simulink library "transformer_lib"  (Simulink 8.1)
settings: Solver=ode45  StartTime=0.0  StopTime=10.0  RelTol=1e-3
undefined symbols (not defined in the file): D1, Delta, Rating, Ts
libraries: powerlib x4, powerlib_extras x2, transformer_lib x1
settings Model: Creator=mi24996  LastModifiedBy=ed12083

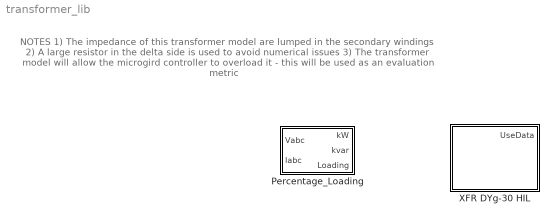
== system transformer_lib ==
  note: NOTES
      | 1) The impedance of this transformer model are lumped in the secondary windings
      | 2) A large resistor in the delta side is used to avoid numerical issues
      | 3) The transformer model will allow the microgird controller to overload it - this will be used as an evaluation metric
  Percentage_Loading : Subsystem  mask(Percentage Loading Block){kVA=Rating}
      mask help:
      | This block calculates the percentage loading of the
      | tranformer in reference to its nameplate data.
  XFR DYg-30 HIL : Subsystem  mask(Transformers){Rating=225, Vp=4160, Vs=208, Z=5.18, XR=2.5}
      mask prompts: Rating "Rating [kVA]"; Vp "Primary Voltage [VRMSLL]"; Vs "Secondary Voltage [VRMSLL]"; Z "Impedance, Z [%]"; XR "X/R Ratio"
      mask help:
      | The distribution transformer is implemented using three single-phase transformers connected D/Ygrounded with a negative 30 degrees angular displacement, and operated with fixed turn ratios.
      | The connectivity convention of this block is as follows: ABC indicates the “primary” or high voltage side, and the abc indicates the “secondary” or low voltage side.

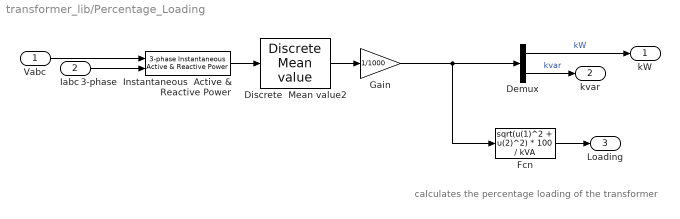
== system transformer_lib/Percentage_Loading ==
  note: calculates the percentage loading of the transformer
  Vabc : Inport
  Iabc : Inport  Port=2
  3-phase  Instantaneous  Active & Reactive Power : powerlib_extras/Measurements/3-phase  Instantaneous  Active & Reactive Power
  Demux : Demux  Outputs=2
  Discrete  Mean value2 : powerlib_extras/Discrete Measurements/Discrete  Mean value  Freq=60  Vinit=0  Ts=Ts
  Fcn : Fcn  Expr=sqrt(u(1)^2 + u(2)^2) * 100 / kVA
  Gain : Gain  Gain=1/1000
  kW : Outport
  kvar : Outport  Port=2
  Loading : Outport  Port=3
  wires:
  Fcn/1 -> Loading/1
  Demux/2 -> kvar/1  "kvar"
  Demux/1 -> kW/1  "kW"
  Iabc/1 -> 3-phase  Instantaneous  Active & Reactive Power/2
  Vabc/1 -> 3-phase  Instantaneous  Active & Reactive Power/1
  Discrete  Mean value2/1 -> Gain/1
  3-phase  Instantaneous  Active & Reactive Power/1 -> Discrete  Mean value2/1
  Gain/1 -> Demux/1, Fcn/1

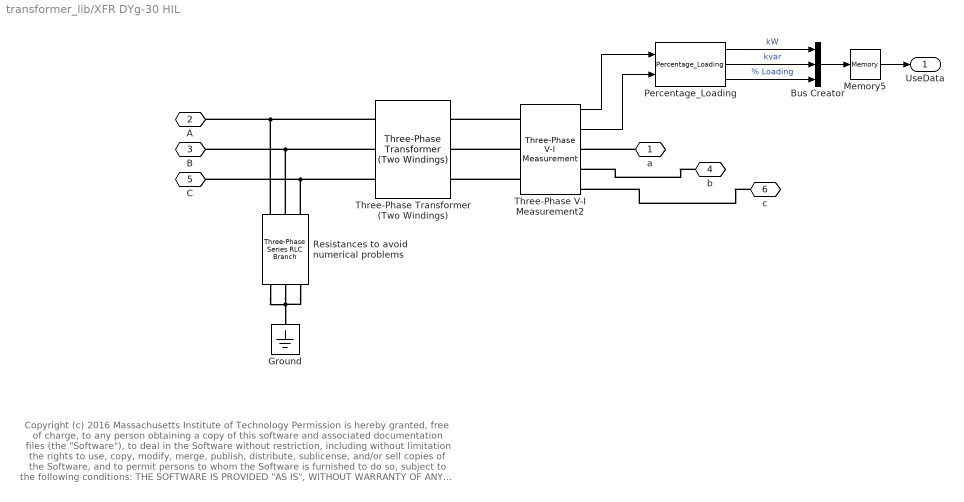
== system transformer_lib/XFR DYg-30 HIL ==
  note: Copyright (c) 2016 Massachusetts Institute of Technology
      | Permission is hereby granted, free of charge, to any person obtaining a copy of this software and associated documentation files (the "Software"), to deal
      | in the Software without restriction, including without limitation the rights to use, copy, modify, merge, publish, distribute, sublicense, and/or sell copies of the
      | Software, and to permit persons to whom the Software is furnished to do so, subject to the following conditions:
      |
      | THE SOFTWARE IS PROVIDED "AS IS", WITHOUT WARRANTY OF ANY KIND, EXPRESS OR IMPLIED, INCLUDING BUT NOT LIMITED TO THE
      | WARRANTIES OF MERCHANTABILITY, FITNESS FOR A PARTICULAR PURPOSE AND NONINFRINGEMENT. IN NO EVENT SHALL THE AUTHORS
      | OR COPYRIGHT HOLDERS BE LIABLE FOR ANY CLAIM, DAMAGES OR OTHER LIABILITY, WHETHER IN AN ACTION OF CONTRACT, TORT OR
      | OTHERWISE, ARISING FROM, OUT OF OR IN CONNECTION WITH THE SOFTWARE OR THE USE OR OTHER DEALINGS IN THE SOFTWARE
  Bus Creator : BusCreator  Inputs=3
  Ground : powerlib/Elements/Ground  LConnTagsString=a
  Memory5 : Memory
  Percentage_Loading : transformer_lib/Percentage_Loading  kVA=Rating
  Resistances to avoid numerical problems : powerlib/Elements/Three-Phase Series RLC Branch  LConnTagsString=A|B|C  RConnTagsString=A|B|C  BranchType=R  Resistance=5e6  Inductance=1e-3  Capacitance=1e-6  Measurements=None
  Three-Phase Transformer (Two Windings) : powerlib/Elements/Three-Phase Transformer (Two Windings)  Winding1Connection=Delta (D1)  UNITS=pu  NominalPower=[ Rating*1E3 , 60 ]  Winding1=[ Vp , 0 , 0]  Winding2Connection=Yg  Winding2=[ Vs , Z/(100*XR) , Z/(2*pi*60*100) ]  SetSaturation=off  Rm=500  Lm=500  Saturation=[ 0,0 ; 0.0024,1.2 ; 1.0,1.52 ]  Hysteresis=off  DataFile='hysteresis'  SetInitialFlux=off  InitialFluxes=[ 0.8 , -0.8 , 0.7 ]  Measurements=None  MoreParameters=off  BreakLoop=off  DataType=off  TransfoNumber=1
  Three-Phase V-I Measurement2 : powerlib/Measurements/Three-Phase V-I Measurement  VoltageMeasurement=phase-to-ground  SetLabelV=off  LabelV=Vabc  Vpu=off  VpuLL=off  CurrentMeasurement=yes  SetLabelI=off  LabelI=Iabc  Ipu=off  Pbase=100e6  Vbase=500e3  OutputType=Complex  PhasorSimulation=off  PSBequivalent=0
  a : PMIOPort  Port=1  Side=Right
  A : PMIOPort  Port=2  Side=Left
  B : PMIOPort  Port=3  Side=Left
  b : PMIOPort  Port=4  Side=Right
  C : PMIOPort  Port=5  Side=Left
  c : PMIOPort  Port=6  Side=Right
  UseData : Outport
  wires:
  Three-Phase V-I Measurement2/2 -> Percentage_Loading/2
  Three-Phase V-I Measurement2/1 -> Percentage_Loading/1
  Percentage_Loading/1 -> Bus Creator/1  "kW"
  Percentage_Loading/2 -> Bus Creator/2  "kvar"
  Percentage_Loading/3 -> Bus Creator/3  "% Loading"
  Bus Creator/1 -> Memory5/1
  Memory5/1 -> UseData/1
  connections:
  Three-Phase Transformer (Two Windings)/LConn3 -- Resistances to avoid numerical problems/LConn3 -- C/RConn1
  Three-Phase Transformer (Two Windings)/LConn2 -- Resistances to avoid numerical problems/LConn2 -- B/RConn1
  Three-Phase Transformer (Two Windings)/LConn1 -- Resistances to avoid numerical problems/LConn1 -- A/RConn1
  Resistances to avoid numerical problems/RConn3 -- Resistances to avoid numerical problems/RConn1 -- Resistances to avoid numerical problems/RConn2 -- Ground/LConn1
  Three-Phase V-I Measurement2/LConn2 -- Three-Phase Transformer (Two Windings)/RConn2
  Three-Phase V-I Measurement2/LConn3 -- Three-Phase Transformer (Two Windings)/RConn3
  Three-Phase V-I Measurement2/LConn1 -- Three-Phase Transformer (Two Windings)/RConn1
  a/RConn1 -- Three-Phase V-I Measurement2/RConn1
  b/RConn1 -- Three-Phase V-I Measurement2/RConn2
  c/RConn1 -- Three-Phase V-I Measurement2/RConn3
